simulink model "springdamper_vector"  (R2022b)
settings: Solver=VariableStepAuto  StartTime=0.0  StopTime=10.0  RelTol=1e-3
settings Model: Creator=a1pab  LastModifiedBy=a1pab

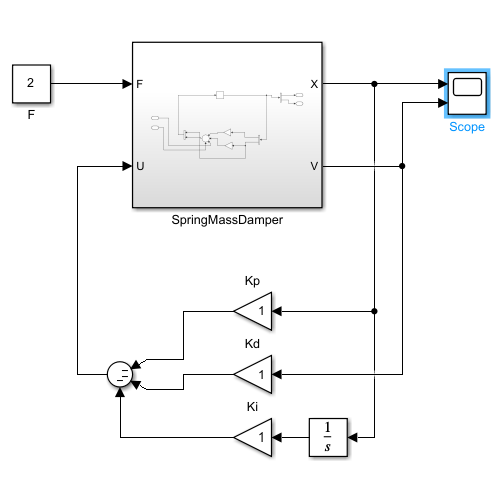
[thumbnail: Simulink's stored preview of the top-level diagram]
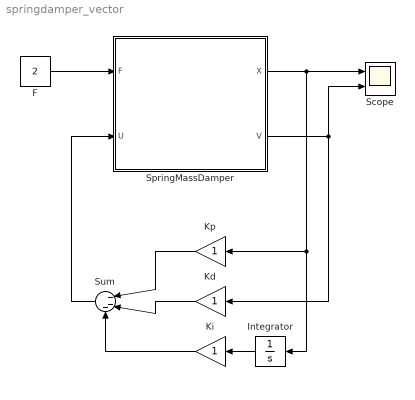
== system springdamper_vector ==
  F : Constant  Value=2
  Integrator : Integrator
  Kd : Gain
  Ki : Gain
  Kp : Gain
  Scope : Scope  NumInputPorts=2
  SpringMassDamper : Subsystem
  Sum : Sum  Inputs=|---
  wires:
  SpringMassDamper/1(X) -> Integrator/1, Kp/1, Scope/1
  F/1 -> SpringMassDamper/1(F)
  SpringMassDamper/2(V) -> Scope/2, Kd/1
  Integrator/1 -> Ki/1
  Kd/1 -> Sum/2
  Kp/1 -> Sum/1
  Ki/1 -> Sum/3
  Sum/1 -> SpringMassDamper/2(U)

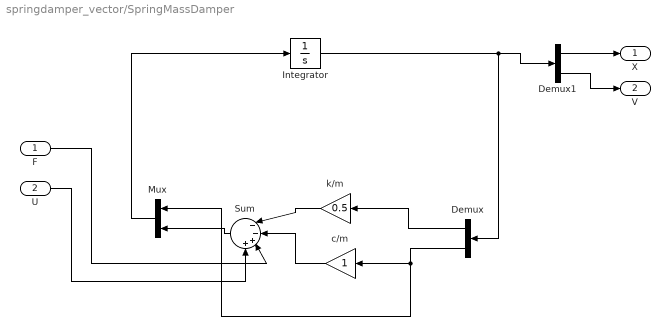
== system springdamper_vector/SpringMassDamper ==
  F : Inport
  U : Inport  Port=2
  Demux : Demux  Outputs=2
  Demux1 : Demux  Outputs=2
  Integrator : Integrator  InitialCondition=[1,0]
  Mux : Mux  Inputs=2
  Sum : Sum  Inputs=|--++
  c/m : Gain
  k/m : Gain  Gain=0.5
  X : Outport
  V : Outport  Port=2
  wires:
  Integrator/1 -> Demux/1, Demux1/1
  Mux/1 -> Integrator/1
  Demux/2 -> Mux/1, c/m/1
  Sum/1 -> Mux/2
  k/m/1 -> Sum/1
  Demux/1 -> k/m/1
  c/m/1 -> Sum/2
  Demux1/1 -> X/1
  Demux1/2 -> V/1
  F/1 -> Sum/3
  U/1 -> Sum/4
